simulink model "testfile_orb_on_PC"  (R2015b)
settings: Solver=VariableStepAuto  StartTime=0.0  StopTime=Inf  RelTol=1e-3
values from neighbouring files (symbols this model uses):
  twist = 0    [plotting_mocap_realsense.m]    (also in plotting_mocap_realsense_orbslam2.m = 1)
undefined symbols (not defined in the file or in its folder): localhost, motion_capture_rate, odom, realsense
libraries: genomix x7
settings Model: Creator=smishra  LastModifiedBy=smishra

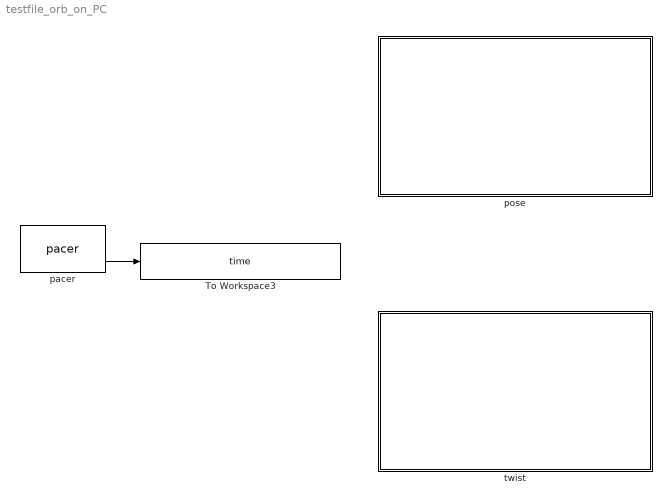
== system testfile_orb_on_PC ==
  To Workspace3 : ToWorkspace  VariableName=time  SampleTime=-1
  pacer : genomix/pacer  Priority=0  catchup=off
  pose : Subsystem
  twist : Subsystem
  wires:
  pacer/2 -> To Workspace3/1

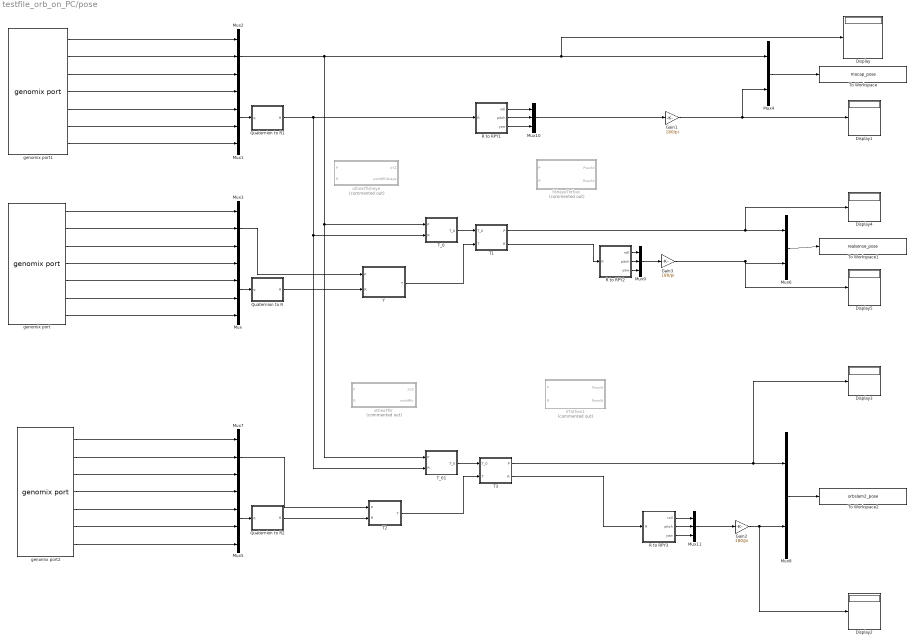
== system testfile_orb_on_PC/pose ==
  Display{,1..5} (6 alike) : Display
  Gain1 : Gain  Gain=180/pi
  Gain2 : Gain  Gain=180/pi
  Gain3 : Gain  Gain=180/pi
  Mux : Mux
  Mux1 : Mux
  Mux{2..3,7,9..11} (6 alike) : Mux  Inputs=3
  Mux4 : Mux  Inputs=2
  Mux5 : Mux
  Mux6 : Mux  Inputs=2
  Mux8 : Mux  Inputs=2
  Quaternion to R : MATLAB Function  SystemSampleTime=motion_capture_rate
  Quaternion to R1 : MATLAB Function  SystemSampleTime=motion_capture_rate
  Quaternion to R2 : MATLAB Function  SystemSampleTime=motion_capture_rate
  R to RPY1 : MATLAB Function  TreatAsAtomicUnit=on
  R to RPY2 : MATLAB Function  TreatAsAtomicUnit=on
  R to RPY3 : MATLAB Function  TreatAsAtomicUnit=on
  T1 : MATLAB Function  SystemSampleTime=motion_capture_rate
  T2 : MATLAB Function  SystemSampleTime=motion_capture_rate
  T3 : MATLAB Function  SystemSampleTime=motion_capture_rate
  T_0 : MATLAB Function  SystemSampleTime=motion_capture_rate
  T_01 : MATLAB Function  SystemSampleTime=motion_capture_rate
  To Workspace : ToWorkspace  VariableName=mocap_pose  SampleTime=-1
  To Workspace1 : ToWorkspace  VariableName=realsense_pose  SampleTime=-1
  To Workspace2 : ToWorkspace  VariableName=orbslam2_pose  SampleTime=-1
  Y : MATLAB Function  SystemSampleTime=motion_capture_rate
  fisheyeTothex : MATLAB Function  Commented=on  SystemSampleTime=motion_capture_rate
  genomix port : genomix/genomix port  host=140.93.16.81:8081  component=manager  port=realsense/odom  sigtype=value  timetype=periodic  period=0.01  siglist="[{\"name\":\"pose.pose.position.x\",\"type\":\"value\",\"size\":1},{\"name\":\"pose.pose.position.y\",\"type\":\"value\",\"size\":1},{\"name\":\"pose.pose.position.z\",\"type\":\"value\",\"size\":1},{\"name\":\"pose.pose.orientation.w\",\"type\":\"value\",\"size\":1},{\"name\":\"pose.pose.orientation.x\",\"type\":\"value\",\"size\":1},{\"name\":\"pose.pose.orientation.y\",\"type\":\"value\",\"size\":1},{\"name\":\"pose.pose.orientation.z\",\"type\":\"value\",\"size\":1}]"
      settings: AttributesFormatString=manager/realsense/odom
  genomix port1 : genomix/genomix port  host=localhost  component=optitrack  port=bodies  subport=OTHex  sigtype=value  timetype=periodic  period=0.01  siglist="[{\"name\":\"bodies.pos.x\",\"type\":\"value\",\"size\":1},{\"name\":\"bodies.pos.y\",\"type\":\"value\",\"size\":1},{\"name\":\"bodies.pos.z\",\"type\":\"value\",\"size\":1},{\"name\":\"bodies.pos.qw\",\"type\":\"value\",\"size\":1},{\"name\":\"bodies.pos.qx\",\"type\":\"value\",\"size\":1},{\"name\":\"bodies.pos.qy\",\"type\":\"value\",\"size\":1},{\"name\":\"bodies.pos.qz\",\"type\":\"value\",\"size\":1}]"
      settings: AttributesFormatString=optitrack/bodies
  genomix port2 : genomix/genomix port  host=localhost:8081  component=ORB_SLAM2  port=pose  sigtype=value  timetype=periodic  period=0.01  siglist="[{\"name\":\"pose.position.x\",\"type\":\"value\",\"size\":1},{\"name\":\"pose.position.y\",\"type\":\"value\",\"size\":1},{\"name\":\"pose.position.z\",\"type\":\"value\",\"size\":1},{\"name\":\"pose.orientation.w\",\"type\":\"value\",\"size\":1},{\"name\":\"pose.orientation.x\",\"type\":\"value\",\"size\":1},{\"name\":\"pose.orientation.y\",\"type\":\"value\",\"size\":1},{\"name\":\"pose.orientation.z\",\"type\":\"value\",\"size\":1}]"
      settings: AttributesFormatString=ORB_SLAM2/pose
  irTothex1 : MATLAB Function  Commented=on  SystemSampleTime=motion_capture_rate
  othexTfiir : MATLAB Function  Commented=on  SystemSampleTime=motion_capture_rate
  othexTfisheye : MATLAB Function  Commented=on  SystemSampleTime=motion_capture_rate
  wires:
  genomix port1/1 -> Mux2/1
  genomix port1/2 -> Mux2/2
  genomix port1/3 -> Mux2/3
  genomix port/2 -> Mux3/2
  genomix port/3 -> Mux3/3
  genomix port/4 -> Mux/1
  genomix port/5 -> Mux/2
  genomix port/6 -> Mux/3
  genomix port/7 -> Mux/4
  Mux/1 -> Quaternion to R/1(q)
  genomix port1/4 -> Mux1/1
  genomix port1/5 -> Mux1/2
  genomix port1/6 -> Mux1/3
  genomix port1/7 -> Mux1/4
  Mux1/1 -> Quaternion to R1/1(q)
  Mux6/1 -> To Workspace1/1
  genomix port/1 -> Mux3/1
  genomix port2/2 -> Mux7/2
  genomix port2/3 -> Mux7/3
  Quaternion to R2/1(R) -> T2/2(R)
  Mux7/1 -> T2/1(P)
  T2/1(T) -> T3/2(T)
  genomix port2/4 -> Mux5/1
  genomix port2/5 -> Mux5/2
  genomix port2/6 -> Mux5/3
  genomix port2/7 -> Mux5/4
  Mux5/1 -> Quaternion to R2/1(q)
  Mux8/1 -> To Workspace2/1
  genomix port2/1 -> Mux7/1
  T_0/1(T_0) -> T1/1(T_0)
  Quaternion to R/1(R) -> Y/2(R)
  Mux3/1 -> Y/1(P)
  Y/1(T) -> T1/2(T)
  T1/1(P) -> Display4/1, Mux6/1
  T1/2(R) -> R to RPY2/1(R)
  R to RPY2/1(roll) -> Mux9/1
  R to RPY2/2(pitch) -> Mux9/2
  R to RPY2/3(yaw) -> Mux9/3
  Mux9/1 -> Gain3/1
  Gain3/1 -> Display5/1, Mux6/2
  Mux4/1 -> To Workspace/1
  R to RPY1/1(roll) -> Mux10/1
  R to RPY1/2(pitch) -> Mux10/2
  R to RPY1/3(yaw) -> Mux10/3
  Gain1/1 -> Mux4/2, Display1/1
  Mux10/1 -> Gain1/1
  Mux2/1 -> Display/1, Mux4/1, T_01/1(P), T_0/1(P)
  Quaternion to R1/1(R) -> T_01/2(R), T_0/2(R), R to RPY1/1(R)
  T_01/1(T_0) -> T3/1(T_0)
  T3/2(R) -> R to RPY3/1(R)
  R to RPY3/1(roll) -> Mux11/1
  R to RPY3/2(pitch) -> Mux11/2
  R to RPY3/3(yaw) -> Mux11/3
  T3/1(P) -> Display3/1, Mux8/1
  Mux11/1 -> Gain2/1
  Gain2/1 -> Display2/1, Mux8/2

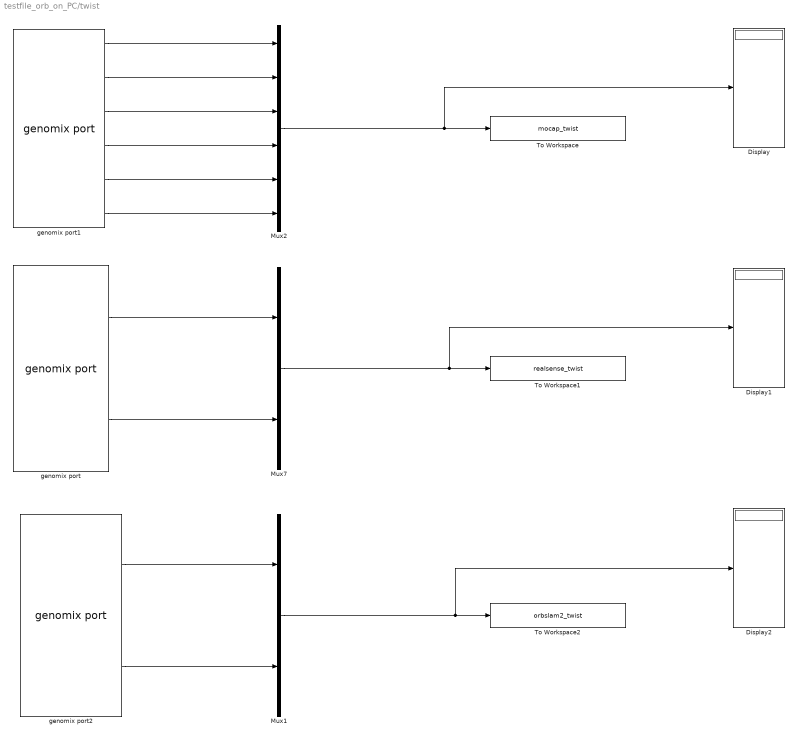
== system testfile_orb_on_PC/twist ==
  Display : Display
  Display1 : Display
  Display2 : Display
  Mux1 : Mux  Inputs=2
  Mux2 : Mux  Inputs=6
  Mux7 : Mux  Inputs=2
  To Workspace : ToWorkspace  VariableName=mocap_twist  SampleTime=-1
  To Workspace1 : ToWorkspace  VariableName=realsense_twist  SampleTime=-1
  To Workspace2 : ToWorkspace  VariableName=orbslam2_twist  SampleTime=-1
  genomix port : genomix/genomix port  host=140.93.16.81:8081  component=manager  port=realsense/odom  sigtype=value  timetype=periodic  period=0.01  siglist="[{\"name\":\"twist.twist.linear\",\"type\":\"value\",\"size\":3},{\"name\":\"twist.twist.angular\",\"type\":\"value\",\"size\":3}]"
      settings: AttributesFormatString=manager/realsense/odom
  genomix port1 : genomix/genomix port  host=localhost  component=pom  port=frame  subport=robot  sigtype=value  timetype=periodic  period=0.01  siglist="[{\"name\":\"frame.vel.vx\",\"type\":\"value\",\"size\":1},{\"name\":\"frame.vel.vy\",\"type\":\"value\",\"size\":1},{\"name\":\"frame.vel.vz\",\"type\":\"value\",\"size\":1},{\"name\":\"frame.vel.wx\",\"type\":\"value\",\"size\":1},{\"name\":\"frame.vel.wy\",\"type\":\"value\",\"size\":1},{\"name\":\"frame.vel.wz\",\"type\":\"value\",\"size\":1}]"
      settings: AttributesFormatString=pom/frame
  genomix port2 : genomix/genomix port  host=localhost:8081  component=ORB_SLAM2  port=odom  sigtype=value  timetype=periodic  period=0.01  siglist="[{\"name\":\"twist.twist.linear\",\"type\":\"value\",\"size\":3},{\"name\":\"twist.twist.angular\",\"type\":\"value\",\"size\":3}]"
      settings: AttributesFormatString=ORB_SLAM2/odom
  wires:
  genomix port1/1 -> Mux2/1
  genomix port1/2 -> Mux2/2
  genomix port1/3 -> Mux2/3
  Mux2/1 -> Display/1, To Workspace/1
  Mux7/1 -> Display1/1, To Workspace1/1
  Mux1/1 -> Display2/1, To Workspace2/1
  genomix port1/4 -> Mux2/4
  genomix port1/5 -> Mux2/5
  genomix port1/6 -> Mux2/6
  genomix port/1 -> Mux7/1
  genomix port/2 -> Mux7/2
  genomix port2/1 -> Mux1/1
  genomix port2/2 -> Mux1/2

== matlab function testfile_orb_on_PC/pose/Quaternion to R1 ==
  data: q input; R output
function R = fcn(q)

R=eye(3);

eta=q(1);
ex=q(2);
ey=q(3);
ez=q(4);

R=[2*(eta^2+ex^2)-1 2*(ex*ey-eta*ez) 2*(ex*ez+eta*ey);
2*(ex*ey+eta*ez) 2*(eta^2+ey^2)-1 2*(ey*ez-eta*ex);
2*(ex*ez-eta*ey) 2*(ey*ez+eta*ex) 2*(eta^2+ez^2)-1];

RCorrect=[1 0 0;0 -1 0; 0 0 -1];
% R=RCorrect*R;

== matlab function testfile_orb_on_PC/pose/R to RPY1 ==
  data: R input; roll output; pitch output; yaw output
function [roll,pitch,yaw] = fcn(R)

roll = atan2(R(3,2),R(3,3));
pitch = atan2(-R(3,1),sqrt(R(3,2)^2+R(3,3)^2));
yaw = atan2(R(2,1),R(1,1));

end

== matlab function testfile_orb_on_PC/pose/T_0 ==
  data: P input; R input; T_0 output
function T_0= fcn(P, R)

P = P(:);

persistent R0 P0

if (isempty(R0) && isempty(P0))
    R0 = R;
    P0 = P;
end

T_0 = [R0 P0; 0 0 0 1];
end

== matlab function testfile_orb_on_PC/pose/Y ==
  data: P input; R input; T output
function T  = fcn(P,R)

T = [R P; 0 0 0 1];

end

== matlab function testfile_orb_on_PC/pose/T1 ==
  data: P output; T_0 input; R output; T input
function [P, R] = fcn(T_0, T)

T = T_0*T;
R = T(1:3,1:3);
P = T(1:3,4);
end

== matlab function testfile_orb_on_PC/pose/R to RPY2 ==
  data: R input; roll output; pitch output; yaw output
function [roll,pitch,yaw] = fcn(R)

roll = atan2(R(3,2),R(3,3));
pitch = atan2(-R(3,1),sqrt(R(3,2)^2+R(3,3)^2));
yaw = atan2(R(2,1),R(1,1));

end

== matlab function testfile_orb_on_PC/pose/othexTfisheye ==
  data: P input; R input; XYZ output; worldRfisheye output
function [XYZ, worldRfisheye]  = fcn(P,R)
% The following is the approximate displacement from the othex origin (IMU) to the euclid's
% fisheye camera origin, measurements done with a simple ruler
% the rotation between the othex frame and the fisheye camera is identity
% x = 2.5 cm;
% y = 4.5 cm;
% z = 6.5 cm;


Tothex = [R P; 0 0 0 1];
othexTfisheye = [eye(3,3) [0.025; 0.045; 0.065]; 0 0 0 1];
T = Tothex * othexTfisheye;

XYZ = T(1:3,4);

worldRfisheye = T(1:3,1:3);
% roll = atan2(worldRfisheye(3,2),worldRfisheye(3,3));
% pitch = atan2(-worldRfisheye(3,1),sqrt(worldRfisheye(3,2)^2+worldRfisheye(3,3)^2));
% yaw = atan2(worldRfisheye(2,1),worldRfisheye(1,1));
% 
% RPY = [roll; pitch; yaw];

end

== matlab function testfile_orb_on_PC/pose/fisheyeTothex ==
  data: P input; R input; Pworld output; Rworld output
function [Pworld, Rworld ]  = fcn(P,R)
% The following is the approximate displacement from the othex origin (IMU) to the euclid's
% fisheye camera origin, measurements done with a simple ruler
% the rotation between the othex frame and the fisheye camera is identity
% x = 2.5 cm;
% y = 4.5 cm;
% z = 6.5 cm;


worldTfisheye = [R P; 0 0 0 1];
othexTfisheye = [eye(3,3) [0.025; 0.045; 0.065]; 0 0 0 1];
fisheyeTothex = inv(othexTfisheye);

worldTothex = worldTfisheye*fisheyeTothex ;

Pworld = worldTothex(1:3,4);
Rworld = worldTothex(1:3,1:3);
end

== matlab function testfile_orb_on_PC/pose/othexTfiir ==
  data: P input; R input; XYZ output; worldRir output
function [XYZ, worldRir]  = fcn(P,R)
% The following is the approximate displacement from the othex origin (IMU) to the euclid's
% left ir camera origin, measurements done with a simple ruler
% the rotation between the othex frame and the left ir camera is identity
% x = 2.5 cm;
% y = 4.5 cm;
% z = 6.5 cm;


Tothex = [R P; 0 0 0 1];
othexTir = [eye(3,3) [0.025; 0.045; 0.065]; 0 0 0 1];
T = Tothex * othexTir;

XYZ = T(1:3,4);

worldRir = T(1:3,1:3);
% roll = atan2(worldRir(3,2),worldRir(3,3));
% pitch = atan2(-worldRir(3,1),sqrt(worldRir(3,2)^2+worldRir(3,3)^2));
% yaw = atan2(worldRir(2,1),worldRir(1,1));
% 
% RPY = [roll; pitch; yaw];

end

== matlab function testfile_orb_on_PC/pose/Quaternion to R2 ==
  data: q input; R output
function R = fcn(q)

R=eye(3);

eta=q(1);
ex=q(2);
ey=q(3);
ez=q(4);

R=[2*(eta^2+ex^2)-1 2*(ex*ey-eta*ez) 2*(ex*ez+eta*ey);
2*(ex*ey+eta*ez) 2*(eta^2+ey^2)-1 2*(ey*ez-eta*ex);
2*(ex*ez-eta*ey) 2*(ey*ez+eta*ex) 2*(eta^2+ez^2)-1];

RCorrect=[1 0 0;0 -1 0; 0 0 -1];
% R=RCorrect*R;

== matlab function testfile_orb_on_PC/pose/R to RPY3 ==
  data: R input; roll output; pitch output; yaw output
function [roll,pitch,yaw] = fcn(R)

roll = atan2(R(3,2),R(3,3));
pitch = atan2(-R(3,1),sqrt(R(3,2)^2+R(3,3)^2));
yaw = atan2(R(2,1),R(1,1));

end

== matlab function testfile_orb_on_PC/pose/T2 ==
  data: P input; R input; T output
function T= fcn(P, R)

T = [R P; 0 0 0 1];

end

== matlab function testfile_orb_on_PC/pose/T3 ==
  data: P output; T_0 input; R output; T input
function [P, R] = fcn(T_0, T)

T = T_0*T;
R = T(1:3,1:3);
P = T(1:3,4);
end

== matlab function testfile_orb_on_PC/pose/irTothex1 ==
  data: P input; R input; Pworld output; Rworld output
function [Pworld, Rworld ]  = fcn(P,R)
% The following is the approximate displacement from the othex origin (IMU) to the euclid's
% ir camera origin, measurements done with a simple ruler
% the rotation between the othex frame and the ir camera is identity
% x = 2.5 cm;
% y = 4.5 cm;
% z = 6.5 cm;


worldTir = [R P; 0 0 0 1];
othexTir = [eye(3,3) [0.025; 0.045; 0.065]; 0 0 0 1];
irTothex = inv(othexTir);

worldTothex = worldTir*irTothex ;

Pworld = worldTothex(1:3,4);
Rworld = worldTothex(1:3,1:3);
end

== matlab function testfile_orb_on_PC/pose/T_01 ==
  data: P input; R input; T_0 output
function T_0= fcn(P, R)

P = P(:);

persistent R0 P0

if (isempty(R0) && isempty(P0))
    R0 = R;
    P0 = P;
end

T_0 = [R0 P0; 0 0 0 1];
end

== matlab function testfile_orb_on_PC/pose/Quaternion to R ==
  data: q input; R output
function R = fcn(q)

R=eye(3);

eta=q(1);
ex=q(2);
ey=q(3);
ez=q(4);

R=[2*(eta^2+ex^2)-1 2*(ex*ey-eta*ez) 2*(ex*ez+eta*ey);
2*(ex*ey+eta*ez) 2*(eta^2+ey^2)-1 2*(ey*ez-eta*ex);
2*(ex*ez-eta*ey) 2*(ey*ez+eta*ex) 2*(eta^2+ez^2)-1];

RCorrect=[1 0 0;0 -1 0; 0 0 -1];
% R=RCorrect*R;
